simulink model "Assignment_2"  (R2020b)
settings: Solver=VariableStepAuto  StartTime=0.0  StopTime=10.0  RelTol=1e-3
undefined symbols (not defined in the file): DiscIntNeverNeededParam
libraries: simulink x1
settings Model: Creator=Shantam Garg  LastModifiedBy=Shantam Garg

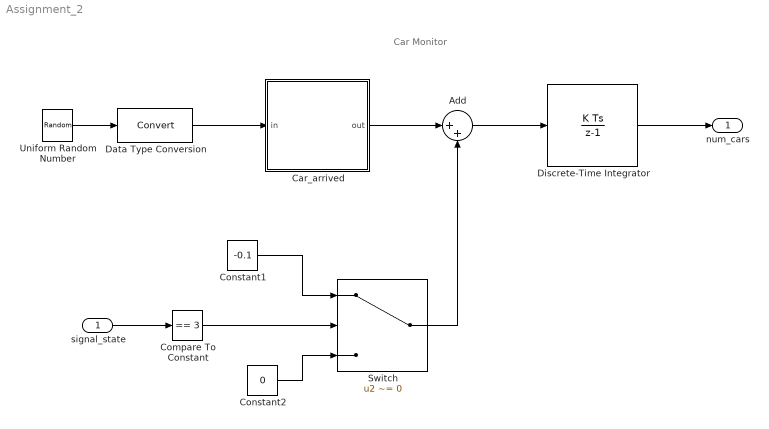
== system Assignment_2 ==
  note: Car Monitor
  signal_state : Inport
  Add : Sum  Inputs=|++
  Car_arrived : Stateflow chart  TreatAsAtomicUnit=on
  Compare To Constant : simulink/Logic and Bit Operations/Compare To Constant  relop===  const=3  OutDataTypeStr=boolean  ZeroCross=off
  Constant1 : Constant  Value=-0.1
  Constant2 : Constant  Value=0
  Data Type Conversion : DataTypeConversion
  Discrete-Time Integrator : DiscreteIntegrator  SampleTime=-1  LimitOutput=on  LowerSaturationLimit=0  ICPrevOutput=DiscIntNeverNeededParam  ICPrevScaledInput=DiscIntNeverNeededParam
  Switch : Switch  Criteria=u2 ~= 0
  Uniform Random Number : UniformRandomNumber  Minimum=0  Maximum=100  Seed=177836  SampleTime=0
  num_cars : Outport  VectorParamsAs1DForOutWhenUnconnected=off
  wires:
  Add/1 -> Discrete-Time Integrator/1
  Compare To Constant/1 -> Switch/2
  signal_state/1 -> Compare To Constant/1
  Constant2/1 -> Switch/3
  Switch/1 -> Add/2
  Car_arrived/1(out) -> Add/1
  Uniform Random Number/1 -> Data Type Conversion/1
  Discrete-Time Integrator/1 -> num_cars/1
  Constant1/1 -> Switch/1
  Data Type Conversion/1 -> Car_arrived/1(in)

== stateflow chart Assignment_2/Car_arrived ==
  (default) -> (junction 2) : {out = in > 98;}
  data: in input int8; out output double
